simulink library "elementsLibrary"  (R2018a)
settings: Solver=VariableStepAuto  StartTime=0.0  StopTime=10.0  RelTol=1e-3
undefined symbols (not defined in the file): aerodynamics, ascent, avionics, environment, payload, propulsion, pvessel, recovery, rocket, sequencer
libraries: snippetLibrary x43, $bdroot x24, sharedutil x8, theirs_elementsLibrary x3, simulink_extras x1, aerolibutil x1
(part 3 of 4)

== system elementsLibrary/Rocktopus/propulsion ==
  time : Inport
  valveCmd : Inport  Port=2
  temp_atm : Inport  Port=3
  pressure_atm : Inport  Port=4
  "density_atm " : Inport  Port=5
  HREV1 : $bdroot/HREV1  propulsion=rocket.propulsion
  gnd{6..9} (4 alike) : Ground
  thrust_B : Outport
  Ve_gas : Outport  Port=2
  propellantMass : Outport  Port=3
  propellantInertias : Outport  Port=4
  engineProperties : Outport  Port=5
  gasExitSpeed : Outport  Port=6
  motorMass : Outport  Port=7
  motorInertias : Outport  Port=8
  motorGeometry : Outport  Port=9
  wires:
  time/1 -> HREV1/1
  valveCmd/1 -> HREV1/2
  temp_atm/1 -> HREV1/3
  pressure_atm/1 -> HREV1/4
  "density_atm "/1 -> HREV1/5
  HREV1/1 -> thrust_B/1
  HREV1/2 -> Ve_gas/1
  HREV1/3 -> propellantMass/1
  HREV1/4 -> propellantInertias/1
  HREV1/5 -> engineProperties/1
  gnd6/1 -> gasExitSpeed/1
  gnd7/1 -> motorMass/1
  gnd8/1 -> motorInertias/1
  gnd9/1 -> motorGeometry/1

== system elementsLibrary/Rocktopus/recovery ==
  windVelocity : Inport
  density_atm : Inport  Port=2
  envConstants : Inport  Port=3
  inQuaternions : Inport  Port=4
  initVelocity_E : Inport  Port=5
  initPosition_E : Inport  Port=6
  inAngVel : Inport  Port=7
  descentOneDeploy : Inport  Port=8
  descentTwoDeploy : Inport  Port=9
  flightState : Inport  Port=10
  SingleChute : $bdroot/SingleChute  recovery=rocket.recovery
  orientationP : Outport
  angularVelocityP : Outport  Port=2
  angularAccelerationP : Outport  Port=3
  angularAccelerationR : Outport  Port=4
  orientationR : Outport  Port=5
  angularVelocityR : Outport  Port=6
  posP_E : Outport  Port=7
  posR_E : Outport  Port=8
  velocityP_E : Outport  Port=9
  velocityR_E : Outport  Port=10
  accelerationR_E : Outport  Port=11
  accelerationP_E : Outport  Port=12
  wires:
  windVelocity/1 -> SingleChute/1
  density_atm/1 -> SingleChute/2
  envConstants/1 -> SingleChute/3
  inQuaternions/1 -> SingleChute/4
  initVelocity_E/1 -> SingleChute/5
  initPosition_E/1 -> SingleChute/6
  inAngVel/1 -> SingleChute/7
  descentOneDeploy/1 -> SingleChute/8
  descentTwoDeploy/1 -> SingleChute/9
  flightState/1 -> SingleChute/10
  SingleChute/1 -> orientationP/1
  SingleChute/2 -> angularVelocityP/1
  SingleChute/3 -> angularAccelerationP/1
  SingleChute/4 -> angularAccelerationR/1
  SingleChute/5 -> orientationR/1
  SingleChute/6 -> angularVelocityR/1
  SingleChute/7 -> posP_E/1
  SingleChute/8 -> posR_E/1
  SingleChute/9 -> velocityP_E/1
  SingleChute/10 -> velocityR_E/1
  SingleChute/11 -> accelerationR_E/1
  SingleChute/12 -> accelerationP_E/1

== system elementsLibrary/Rocktopus/sequencer ==
  position_E : Inport
  orientation : Inport  Port=2
  velocity_E : Inport  Port=3
  thrust_B : Inport  Port=4
  descentOneDeploy : Inport  Port=5
  descentTwoDeploy : Inport  Port=6
  FSv1 : $bdroot/FSv1  sequencer=rocket.sequencer
  flightState : Outport
  towerVector : Outport  Port=2
  wires:
  position_E/1 -> FSv1/1
  orientation/1 -> FSv1/2
  velocity_E/1 -> FSv1/3
  thrust_B/1 -> FSv1/4
  descentOneDeploy/1 -> FSv1/5
  descentTwoDeploy/1 -> FSv1/6
  FSv1/1 -> flightState/1
  FSv1/2 -> towerVector/1

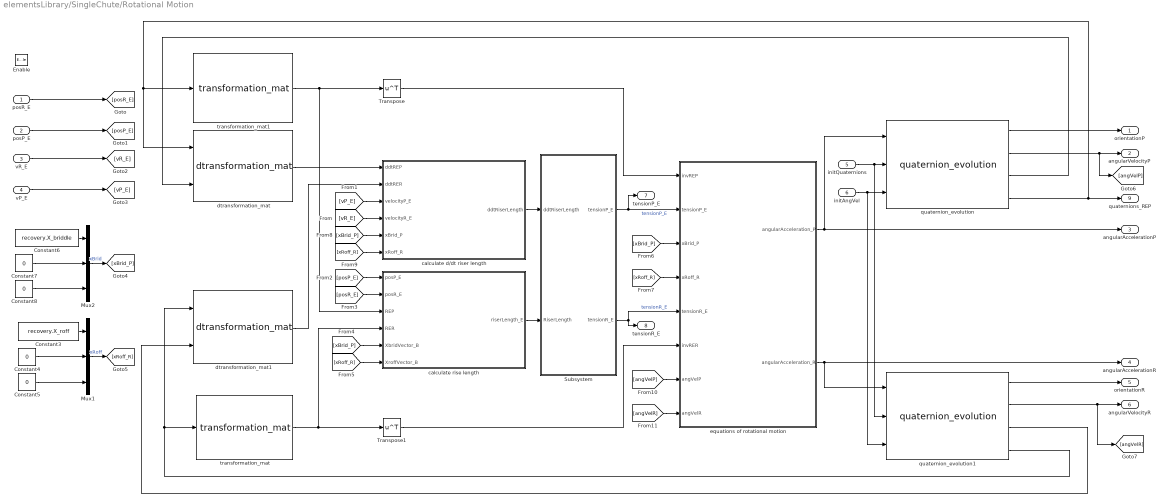
== system elementsLibrary/SingleChute/Rotational Motion ==
  posR_E : Inport
  posP_E : Inport  Port=2
  vR_E : Inport  Port=3
  vP_E : Inport  Port=4
  initQuaternions : Inport  Port=5
  initAngVel : Inport  Port=6
  Enable : EnablePort  StatesWhenEnabling=reset
  Constant3 : Constant  Value=recovery.X_roff
  Constant{4..5,7..8} (4 alike) : Constant  Value=0
  Constant6 : Constant  Value=recovery.X_briddle
  Mux1 : Mux  Inputs=3
  Mux2 : Mux  Inputs=3
  Subsystem : Subsystem
  Transpose : Math  Operator=transpose  SaturateOnIntegerOverflow=on
  Transpose1 : Math  Operator=transpose  SaturateOnIntegerOverflow=on
  calculate d/dt riser length : Subsystem
  calculate rise length : Subsystem
  dtransformation_mat : snippetLibrary/mathSnippets/dtransformation_mat
  dtransformation_mat1 : snippetLibrary/mathSnippets/dtransformation_mat
  equations of rotational motion : Subsystem
  quaternion_evolution : snippetLibrary/mathSnippets/quaternion_evolution
  quaternion_evolution1 : snippetLibrary/mathSnippets/quaternion_evolution
  transformation_mat : snippetLibrary/mathSnippets/transformation_mat
  transformation_mat1 : snippetLibrary/mathSnippets/transformation_mat
  orientationP : Outport
  angularVelocityP : Outport  Port=2
  angularAccelerationP : Outport  Port=3
  angularAccelerationR : Outport  Port=4
  orientationR : Outport  Port=5
  angularVelocityR : Outport  Port=6
  tensionP_E : Outport  Port=7
  tensionR_E : Outport  Port=8
  quaternions_REP : Outport  Port=9
  wires:
  [xRoff_R] -> calculate rise length/6(XroffVector_B)
  equations of rotational motion/2(angularAcceleration_R) -> angularAccelerationR/1, quaternion_evolution1/1
  [posR_E] -> calculate rise length/2(posR_E)
  [posP_E] -> calculate rise length/1(posP_E)
  Constant4/1 -> Mux1/2
  Mux1/1 -> [xRoff_R]  "xRoff"
  posP_E/1 -> [posP_E]
  Subsystem/1(tensionP_E) -> tensionP_E/1, equations of rotational motion/2(tensionP_E)  "tensionP_E"
  calculate d/dt riser length/1(ddtRiserLength) -> Subsystem/1(ddtRiserLength)
  Constant6/1 -> Mux2/1
  calculate rise length/1(riserLength_E) -> Subsystem/2(RiserLength)
  posR_E/1 -> [posR_E]
  [xBrid_P] -> equations of rotational motion/3(xBrid_P)
  [xRoff_R] -> equations of rotational motion/4(xRoff_R)
  [vR_E] -> calculate d/dt riser length/4(velocityR_E)
  Transpose/1 -> equations of rotational motion/1(invREP)
  vP_E/1 -> [vP_E]
  equations of rotational motion/1(angularAcceleration_P) -> angularAccelerationP/1, quaternion_evolution/1
  vR_E/1 -> [vR_E]
  Mux2/1 -> [xBrid_P]  "xBrid"
  Subsystem/2(tensionR_E) -> tensionR_E/1, equations of rotational motion/5(tensionR_E)  "tensionR_E"
  Constant8/1 -> Mux2/3
  Constant3/1 -> Mux1/1
  Constant7/1 -> Mux2/2
  Constant5/1 -> Mux1/3
  [xBrid_P] -> calculate rise length/5(XbridVector_B)
  [vP_E] -> calculate d/dt riser length/3(velocityP_E)
  Transpose1/1 -> equations of rotational motion/6(invRER)
  quaternion_evolution/2 -> angularVelocityP/1, [angVelP]
  quaternion_evolution/1 -> orientationP/1
  quaternion_evolution1/1 -> orientationR/1
  quaternion_evolution1/2 -> [angVelR], angularVelocityR/1
  dtransformation_mat/1 -> calculate d/dt riser length/1(ddtREP)
  transformation_mat1/1 -> Transpose/1, calculate rise length/3(REP)
  transformation_mat/1 -> Transpose1/1, calculate rise length/4(RER)
  quaternion_evolution1/3 -> dtransformation_mat1/2
  quaternion_evolution/3 -> dtransformation_mat/2
  quaternion_evolution1/4 -> transformation_mat/1, dtransformation_mat1/1
  quaternion_evolution/4 -> quaternions_REP/1, transformation_mat1/1, dtransformation_mat/1
  dtransformation_mat1/1 -> calculate d/dt riser length/2(ddtRER)
  [xBrid_P] -> calculate d/dt riser length/5(xBrid_P)
  [xRoff_R] -> calculate d/dt riser length/6(xRoff_R)
  initQuaternions/1 -> quaternion_evolution1/2, quaternion_evolution/2
  [angVelP] -> equations of rotational motion/7(angVelP)
  [angVelR] -> equations of rotational motion/8(angVelR)
  initAngVel/1 -> quaternion_evolution/3, quaternion_evolution1/3

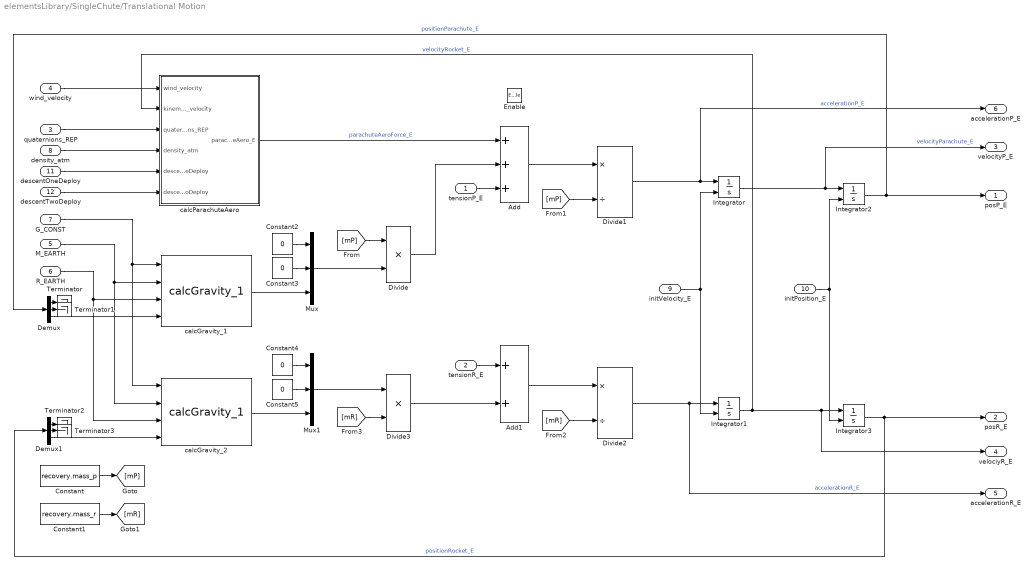
== system elementsLibrary/SingleChute/Translational Motion ==
  tensionP_E : Inport
  tensionR_E : Inport  Port=2
  quaternions_REP : Inport  Port=3
  wind_velocity : Inport  Port=4
  M_EARTH : Inport  Port=5
  R_EARTH : Inport  Port=6
  G_CONST : Inport  Port=7
  density_atm : Inport  Port=8
  initVelocity_E : Inport  Port=9
  initPosition_E : Inport  Port=10
  descentOneDeploy : Inport  Port=11
  descentTwoDeploy : Inport  Port=12
  Enable : EnablePort  StatesWhenEnabling=reset
  Add : Sum  Inputs=+++
  Add1 : Sum
  Constant : Constant  Value=recovery.mass_p
  Constant1 : Constant  Value=recovery.mass_r
  Constant{2..5} (4 alike) : Constant  Value=0
  Demux : Demux  Outputs=3
  Demux1 : Demux  Outputs=3
  Divide : Product  Inputs=**
  Divide1 : Product  Inputs=*/
  Divide2 : Product  Inputs=*/
  Divide3 : Product  Inputs=**
  Integrator{,1..3} (4 alike) : Integrator  InitialConditionSource=external
  Mux : Mux  Inputs=3
  Mux1 : Mux  Inputs=3
  Terminator{,1..3} (4 alike) : Terminator
  calcGravity_1 : snippetLibrary/dynamicsSnippets/calcGravity_1
  calcGravity_2 : snippetLibrary/dynamicsSnippets/calcGravity_1
  "calcParachuteAero " : Subsystem
  posP_E : Outport
  posR_E : Outport  Port=2
  velocityP_E : Outport  Port=3
  velociyR_E : Outport  Port=4
  accelerationR_E : Outport  Port=5
  accelerationP_E : Outport  Port=6
  wires:
  Add1/1 -> Divide2/1
  tensionP_E/1 -> Add/3
  Divide1/1 -> accelerationP_E/1, Integrator/1  "accelerationP_E"
  Integrator/1 -> velocityP_E/1, Integrator2/1  "velocityParachute_E"
  [mP] -> Divide1/2
  Divide2/1 -> accelerationR_E/1, Integrator1/1  "accelerationR_E"
  tensionR_E/1 -> Add1/1
  Add/1 -> Divide1/1
  Constant/1 -> [mP]
  "calcParachuteAero "/1(parachuteAero_E) -> Add/1  "parachuteAeroForce_E"
  [mR] -> Divide2/2
  Divide/1 -> Add/2
  Integrator1/1 -> velociyR_E/1, Integrator3/1, "calcParachuteAero "/2(kinematic_velocity)  "velocityRocket_E"
  Constant1/1 -> [mR]
  Integrator2/1 -> Demux/1, posP_E/1  "positionParachute_E"
  Integrator3/1 -> Demux1/1, posR_E/1  "positionRocket_E"
  quaternions_REP/1 -> "calcParachuteAero "/3(quaternions_REP)
  wind_velocity/1 -> "calcParachuteAero "/1(wind_velocity)
  Divide3/1 -> Add1/2
  [mR] -> Divide3/2
  [mP] -> Divide/1
  Constant2/1 -> Mux/1
  Constant3/1 -> Mux/2
  calcGravity_1/1 -> Mux/3
  Mux/1 -> Divide/2
  calcGravity_2/1 -> Mux1/3
  Mux1/1 -> Divide3/1
  Constant4/1 -> Mux1/1
  Constant5/1 -> Mux1/2
  R_EARTH/1 -> calcGravity_1/3, calcGravity_2/3
  M_EARTH/1 -> calcGravity_1/2, calcGravity_2/2
  G_CONST/1 -> calcGravity_1/1, calcGravity_2/1
  density_atm/1 -> "calcParachuteAero "/4(density_atm)
  Demux/3 -> calcGravity_1/4
  Demux1/3 -> calcGravity_2/4
  initVelocity_E/1 -> Integrator1/2, Integrator/2
  initPosition_E/1 -> Integrator2/2, Integrator3/2
  descentOneDeploy/1 -> "calcParachuteAero "/5(descentOneDeploy)
  descentTwoDeploy/1 -> "calcParachuteAero "/6(descentTwoDeploy)
  Demux1/1 -> Terminator2/1
  Demux1/2 -> Terminator3/1
  Demux/1 -> Terminator/1
  Demux/2 -> Terminator1/1

== system elementsLibrary/SolidMotor/calculate motor inertia ==
  motorMass : Inport
  grainInnerDia : Inport  Port=2
  grainOuterDia : Inport  Port=3
  grainLength : Inport  Port=4
  Add : Sum
  Add1 : Sum
  Constant{,1..5} (6 alike) : Constant  Value=0
  Create 3x3 Matrix : sharedutil/Create 3x3 Matrix  aMode=aMode
  Gain : Gain  Gain=0.5
  Gain1 : Gain  Gain=0.5
  Gain2 : Gain  Gain=3
  Gain3 : Gain  Gain=1/12
  Gain4 : Gain  Gain=0.5
  Gain5 : Gain
  Multiply : Product
  Multiply1 : Product
  Square : Math  Operator=square  SaturateOnIntegerOverflow=on
  Square1 : Math  Operator=square  SaturateOnIntegerOverflow=on
  Square2 : Math  Operator=square  SaturateOnIntegerOverflow=on
  J_motor : Outport
  wires:
  Create 3x3 Matrix/1 -> J_motor/1  "inertias"
  grainLength/1 -> Square2/1
  grainInnerDia/1 -> Gain/1
  Gain/1 -> Square/1
  grainOuterDia/1 -> Gain1/1
  Gain1/1 -> Square1/1
  Square/1 -> Add/1
  Square1/1 -> Add/2
  Add/1 -> Multiply1/1, Gain2/1
  Gain2/1 -> Add1/1
  Square2/1 -> Add1/2
  motorMass/1 -> Gain3/1
  Add1/1 -> Multiply/1
  Gain3/1 -> Multiply1/2, Multiply/2
  Multiply/1 -> Create 3x3 Matrix/9, Gain5/1  "Izz"
  Multiply1/1 -> Gain4/1
  Gain4/1 -> Create 3x3 Matrix/1  "Ixx"
  Gain5/1 -> Create 3x3 Matrix/5  "Iyy"
  Constant/1 -> Create 3x3 Matrix/2
  Constant1/1 -> Create 3x3 Matrix/3
  Constant2/1 -> Create 3x3 Matrix/4
  Constant3/1 -> Create 3x3 Matrix/6
  Constant4/1 -> Create 3x3 Matrix/7
  Constant5/1 -> Create 3x3 Matrix/8

== system elementsLibrary/barrowmanExt/CalcMach ==
  Temperatue_atm : Inport
  kinematicVelocity : Inport  Port=2
  Add : Sum
  Constant : Constant  Value=20.05
  Constant1 : Constant  Value=273.1
  Divide : Product  Inputs=*/
  Multiply : Product
  Sqrt : Sqrt  SaturateOnIntegerOverflow=on
  magnitude_3 : snippetLibrary/mathSnippets/magnitude_3
  Mach : Outport
  wires:
  Temperatue_atm/1 -> Add/2
  Constant1/1 -> Add/1
  Add/1 -> Sqrt/1
  Constant/1 -> Multiply/2
  Sqrt/1 -> Multiply/1
  Multiply/1 -> Divide/2
  Divide/1 -> Mach/1
  kinematicVelocity/1 -> magnitude_3/1
  magnitude_3/1 -> Divide/1

== system elementsLibrary/barrowmanExt/Center of Pressure ==
  Cna_body : Inport
  Cna_fins : Inport  Port=2
  Cna_nosecone : Inport  Port=3
  Mach : Inport  Port=4
  Add : Sum  Inputs=+++
  Add1 : Sum  Inputs=+++
  Calc Xcp fins : Subsystem
  Constant : Constant  Value=aerodynamics.Xcp_nose
  Constant2 : Constant  Value=aerodynamics.Xcp_body
  Divide : Product  Inputs=*/
  Multiply : Product
  Multiply1 : Product
  Multiply2 : Product
  Xcp : Outport
  wires:
  Constant/1 -> Multiply/2
  Cna_nosecone/1 -> Add1/3, Multiply/1
  Cna_fins/1 -> Add1/2, Multiply2/1
  Constant2/1 -> Multiply1/1
  Cna_body/1 -> Add1/1, Multiply1/2
  Multiply/1 -> Add/3
  Multiply2/1 -> Add/2
  Multiply1/1 -> Add/1
  Add/1 -> Divide/1
  Add1/1 -> Divide/2
  Divide/1 -> Xcp/1
  Calc Xcp fins/1(Xcp_fins) -> Multiply2/2
  Mach/1 -> Calc Xcp fins/1(Mach)

== system elementsLibrary/barrowmanExt/Coeff multiplier ==
  Velocity_B : Inport
  Density_air : Inport  Port=2
  Constant : Constant  Value=0.5
  Constant1 : Constant  Value=aerodynamics.Ar
  Multiply : Product  Inputs=4
  Square : Math  Operator=square  SaturateOnIntegerOverflow=on
  magnitude_3 : Subsystem
  Coeff_mul : Outport
  wires:
  Velocity_B/1 -> magnitude_3/1(vector)
  magnitude_3/1(magnitude) -> Square/1
  Square/1 -> Multiply/1
  Density_air/1 -> Multiply/2
  Constant/1 -> Multiply/3
  Constant1/1 -> Multiply/4
  Multiply/1 -> Coeff_mul/1

== system elementsLibrary/barrowmanExt/Coeff multiplier1 ==
  Velocity_B : Inport
  Density_air : Inport  Port=2
  Constant : Constant  Value=0.5
  Constant1 : Constant  Value=aerodynamics.Ar
  Constant2 : Constant  Value=aerodynamics.dn
  Multiply : Product  Inputs=5
  Square : Math  Operator=square  SaturateOnIntegerOverflow=on
  magnitude_3 : Subsystem
  Coeff_mul : Outport
  wires:
  Velocity_B/1 -> magnitude_3/1(vector)
  magnitude_3/1(magnitude) -> Square/1
  Square/1 -> Multiply/1
  Density_air/1 -> Multiply/2
  Constant/1 -> Multiply/3
  Constant1/1 -> Multiply/4
  Multiply/1 -> Coeff_mul/1
  Constant2/1 -> Multiply/5

== system elementsLibrary/barrowmanExt/Coefficent of drag 0 AOA ==
  Mach : Inport
  RE_Body : Inport  Port=2
  RE_Fins : Inport  Port=3
  Add : Sum  Inputs=+++
  Base Drag Coefficient : Subsystem
  Friction Drag Coefficient : Subsystem
  Pressure Drag Coefficient : Subsystem
  Cd_0 : Outport
  wires:
  RE_Body/1 -> Friction Drag Coefficient/2(RE_Body)
  RE_Fins/1 -> Friction Drag Coefficient/3(RE_Fins)
  Mach/1 -> Pressure Drag Coefficient/2(mach), Friction Drag Coefficient/1(mach), Base Drag Coefficient/1(Mach)
  Base Drag Coefficient/1(Cd_Base) -> Add/1, Pressure Drag Coefficient/1(Cd_Base)
  Pressure Drag Coefficient/1(Cd_Pressure) -> Add/2
  Friction Drag Coefficient/1(CD_Friction) -> Add/3
  Add/1 -> Cd_0/1

== system elementsLibrary/barrowmanExt/Coefficient of Axial Force ==
  AOA : Inport
  Cd_0 : Inport  Port=2
  If : If  IfExpression=u1 <=0.2967
  If Action Subsystem : Subsystem  TreatAsAtomicUnit=on
  If Action Subsystem1 : Subsystem  TreatAsAtomicUnit=on
  If Action Subsystem2 : Subsystem  TreatAsAtomicUnit=on
  If Action Subsystem3 : Subsystem  TreatAsAtomicUnit=on
  If Action Subsystem4 : Subsystem  TreatAsAtomicUnit=on
  If Action Subsystem5 : Subsystem  TreatAsAtomicUnit=on
  If1 : If  IfExpression=u1 > 1.5708
  If2 : If  IfExpression=u1 > 1.5708
  Merge : Merge
  Merge1 : Merge
  Merge2 : Merge
  Multiply : Product
  Cax : Outport
  wires:
  If/1 -> If Action Subsystem/Action
  AOA/1 -> If2/1, If Action Subsystem2/1(AOA_init), If Action Subsystem1/1(AOA_init), If1/1
  If1/1 -> If Action Subsystem1/Action
  If1/2 -> If Action Subsystem2/Action
  If Action Subsystem2/1(AOA) -> Merge/2
  If Action Subsystem1/1(AOA) -> Merge/1
  Merge/1 -> If Action Subsystem3/1(AOA), If/1, If Action Subsystem/1(AOA)
  If/2 -> If Action Subsystem3/Action
  If Action Subsystem/1(Ax_multi) -> Merge1/1
  If Action Subsystem3/1(Ax_multi) -> Merge1/2
  If2/1 -> If Action Subsystem4/Action
  If2/2 -> If Action Subsystem5/Action
  Merge1/1 -> If Action Subsystem4/1(Ax_multi_init), If Action Subsystem5/1(Ax_multi_init)
  If Action Subsystem4/1(Ax_multi) -> Merge2/1
  If Action Subsystem5/1(Ax_multi) -> Merge2/2
  Merge2/1 -> Multiply/2
  Cd_0/1 -> Multiply/1
  Multiply/1 -> Cax/1

== system elementsLibrary/barrowmanExt/Coefficient of normal force ==
  k1 : Inport
  k2 : Inport  Port=2
  k3 : Inport  Port=3
  Mach : Inport  Port=4
  AOA : Inport  Port=5
  Add : Sum
  Add1 : Sum
  Body tube correction : Subsystem
  Cna Body Tube : Subsystem
  Cna Fins : Subsystem
  Divide : Product  Inputs=*/
  Multiply : Product
  Cn : Outport
  Cna_body : Outport  Port=2
  Cna_fins : Outport  Port=3
  Cna_nosecone : Outport  Port=4
  wires:
  AOA/1 -> Cna Fins/1(AOA), Body tube correction/1(AOA), Divide/2, Multiply/1, Cna Body Tube/1(AOA)
  Mach/1 -> Cna Fins/2(Mach)
  k1/1 -> Cna Fins/3(k1)
  k2/1 -> Cna Fins/4(k2)
  k3/1 -> Cna Fins/5(k3)
  Cna Body Tube/1(Cna_nosecone) -> Cna_nosecone/1, Add/1
  Cna Fins/1(Cna_fins_w_FB_inter) -> Cna_fins/1, Add/2
  Add/1 -> Multiply/2
  Body tube correction/1(Cn_BodyCorrection) -> Divide/1, Add1/1
  Multiply/1 -> Add1/2
  Add1/1 -> Cn/1
  Divide/1 -> Cna_body/1

== system elementsLibrary/barrowmanExt/Moment Coefficients from nosetip ==
  Xcp : Inport
  Cn : Inport  Port=2
  rollAngle : Inport  Port=3
  Xcg : Inport  Port=4
  Constant1 : Constant  Value=0
  Cos : Trigonometry  Operator=cos
  Multiply : Product
  Multiply1 : Product
  Pitch Moment Coeff : Subsystem
  Sin : Trigonometry
  Subsystem : Subsystem
  Cm_roll : Outport
  Cm_pitch : Outport  Port=2
  Cm_yaw : Outport  Port=3
  wires:
  Xcp/1 -> Pitch Moment Coeff/1(Xcp)
  Cn/1 -> Subsystem/2(Cn), Pitch Moment Coeff/2(Cn)
  Pitch Moment Coeff/1(Cm_pitch_cp) -> Subsystem/1(Cm_pitch_cp)
  Xcg/1 -> Subsystem/3(Xcg)
  Cos/1 -> Multiply/1
  Multiply1/1 -> Cm_yaw/1
  Multiply/1 -> Cm_pitch/1
  rollAngle/1 -> Cos/1, Sin/1
  Subsystem/1(Cm_pitch_cg) -> Multiply1/1, Multiply/2
  Sin/1 -> Multiply1/2
  Constant1/1 -> Cm_roll/1

== system elementsLibrary/barrowmanExt/Reynolds num ==
  Velocity : Inport
  Kinematic Viscosity : Inport  Port=2
  Constant : Constant  Value=aerodynamics.l_TR
  Constant1 : Constant  Value=aerodynamics.lm
  Divide : Product  Inputs=*/
  Multiply : Product
  Multiply1 : Product
  magnitude_3 : snippetLibrary/mathSnippets/magnitude_3
  Reynolds_Body : Outport
  Reynolds_Fins : Outport  Port=2
  wires:
  Kinematic Viscosity/1 -> Divide/2
  Multiply/1 -> Reynolds_Body/1
  Constant/1 -> Multiply/1
  Divide/1 -> Multiply1/1, Multiply/2
  Multiply1/1 -> Reynolds_Fins/1
  Constant1/1 -> Multiply1/2
  Velocity/1 -> magnitude_3/1
  magnitude_3/1 -> Divide/1

== system elementsLibrary/nitrousTank1/Nitrous_Inertia_and_cg ==
  mass : Inport
  density : Inport  Port=2
  Add : Sum
  Constant{,1..6} (7 alike) : Constant  Value=0
  Constant10 : Constant  Value=pvessel.L_OxiTank
  Constant7 : Constant  Value=pi
  Constant8 : Constant  Value=2
  Constant9 : Constant  Value=pvessel.D_OxiTank
  Create 3x3 Matrix : sharedutil/Create 3x3 Matrix  aMode=aMode
  Divide : Product  Inputs=*/
  Divide1 : Product  Inputs=*/
  Divide2 : Product  Inputs=*/
  Gain : Gain  Gain=1/12
  Gain1 : Gain  Gain=1/2
  Gain2 : Gain  Gain=3
  Gain3 : Gain  Gain=1/2
  Multiply : Product
  Multiply1 : Product
  Square : Math  Operator=square  SaturateOnIntegerOverflow=on
  Square1 : Math  Operator=square  SaturateOnIntegerOverflow=on
  Square2 : Math  Operator=square  SaturateOnIntegerOverflow=on
  Terminator : Terminator
  Inertia_oxi : Outport
  X_cg : Outport  Port=2
  wires:
  Constant9/1 -> Gain3/1, Gain1/1
  Gain1/1 -> Square1/1
  Square1/1 -> Gain2/1
  Square/1 -> Add/1
  Gain2/1 -> Add/2
  Gain/1 -> Multiply/1
  Add/1 -> Multiply/2
  Multiply/1 -> Create 3x3 Matrix/4, Create 3x3 Matrix/9
  Constant/1 -> Create 3x3 Matrix/2
  Constant1/1 -> Create 3x3 Matrix/1
  Constant2/1 -> Create 3x3 Matrix/3
  Constant3/1 -> Create 3x3 Matrix/5
  Constant4/1 -> Create 3x3 Matrix/6
  Constant5/1 -> Create 3x3 Matrix/7
  Constant6/1 -> Create 3x3 Matrix/8
  Create 3x3 Matrix/1 -> Inertia_oxi/1
  Gain3/1 -> Square2/1  "r_oxi"
  Square2/1 -> Multiply1/2
  Divide2/1 -> Divide/1, Square/1  "h_oxi"
  Constant8/1 -> Divide/2
  Divide1/1 -> Divide2/1  "Volume_oxi"
  density/1 -> Divide1/2
  mass/1 -> Divide1/1, Gain/1  "mass_oxi"
  Multiply1/1 -> Divide2/2  "Pi*(r2)"
  Constant7/1 -> Multiply1/1
  Divide/1 -> X_cg/1
  Constant10/1 -> Terminator/1

== system elementsLibrary/Ascentv1/Calculate Aero Coeffs & Center of Pressure/calculate AOA & Side Slip ==
  apparentVelocity_B : Inport
  calcAoA : MATLAB Function  TreatAsAtomicUnit=on
  AOA : Outport
  aeroRollAngle : Outport  Port=2
  wires:
  calcAoA/1(alpha) -> AOA/1
  apparentVelocity_B/1 -> calcAoA/1(Va)
  calcAoA/2(phiA) -> aeroRollAngle/1

== system elementsLibrary/Ascentv1/Calculate Aero Coeffs & Center of Pressure/calculate Mach ==
  temperature_atm : Inport
  apparentVelocity_E : Inport  Port=2
  Add : Sum
  Constant : Constant  Value=331.3
  Constant1 : Constant  Value=0.606
  Divide : Product  Inputs=*/
  Multiply : Product
  magnitude_3 : snippetLibrary/mathSnippets/magnitude_3
  mach : Outport
  speed of sound : Outport  Port=2
  wires:
  Constant1/1 -> Multiply/2
  Multiply/1 -> Add/1
  Constant/1 -> Add/2
  Add/1 -> Divide/2, speed of sound/1  "speedOfSound"
  Divide/1 -> mach/1  "mach"
  apparentVelocity_E/1 -> magnitude_3/1
  magnitude_3/1 -> Divide/1  "VaMag_B"
  temperature_atm/1 -> Multiply/1

== system elementsLibrary/Ascentv1/Calculate Aero Coeffs & Center of Pressure/calculate ZAOA_cd ==
  note: Calculating Relavent Reynolds Number
  apparentVelocity_B : Inport
  density_atm : Inport  Port=2
  kinViscosity_atm : Inport  Port=3
  Add : Sum  Inputs=++++
  BaseCd : Subsystem
  Constant : Constant  Value=ascent.aerodynamics.l_TR
  Constant1 : Constant  Value=ascent.aerodynamics.lm
  Constant2 : Constant  Value=ascent.aerodynamics.REC
  Divide : Product  Inputs=*/
  FinsetCd : Subsystem
  ForebodyCd : Subsystem
  InterferenceCd : Subsystem
  MATLAB Function : snippetLibrary/aeroSnippets/MATLAB Function
  MATLAB Function1 : snippetLibrary/aeroSnippets/MATLAB Function
  Multiply1 : Product
  Multiply2 : Product
  Terminator : Terminator
  magnitude_3 : snippetLibrary/mathSnippets/magnitude_3
  ZAOA_cd : Outport
  wires:
  magnitude_3/1 -> Divide/1
  Divide/1 -> Multiply1/2, Multiply2/1
  Constant/1 -> Multiply1/1
  Constant1/1 -> Multiply2/2
  Multiply1/1 -> MATLAB Function/1  "reynoldBody"
  Multiply2/1 -> MATLAB Function1/1  "reynoldFinSet"
  Constant2/1 -> MATLAB Function1/2, MATLAB Function/2
  MATLAB Function/1 -> ForebodyCd/1(Cf_fb)  "cf_fb"
  MATLAB Function1/1 -> InterferenceCd/1(Cf_f), FinsetCd/1(Cf_f)  "cf_f"
  FinsetCd/1(Cdf) -> Add/4  "Cdf"
  Add/1 -> ZAOA_cd/1  "ZAOA_cd"
  ForebodyCd/1(Cd_fb) -> Add/1, BaseCd/1(Cd_fb)  "Cd_fb"
  BaseCd/1(Cdb) -> Add/2
  InterferenceCd/1(Cdi) -> Add/3  "Cdi"
  kinViscosity_atm/1 -> Divide/2
  apparentVelocity_B/1 -> magnitude_3/1
  density_atm/1 -> Terminator/1

== system elementsLibrary/Ascentv1/Rotation/Subsystem ==
  angVel : Inport
  sumOfMoments : Inport  Port=2
  J_rocket : Inport  Port=3
  Add : Sum  Inputs=-+
  Matrix Multiply : Product  Inputs=/*  Multiplication=Matrix(*)
  Matrix Multiply2 : Product  Multiplication=Matrix(*)
  crossProduct : snippetLibrary/mathSnippets/crossProduct
  angularAcceleration : Outport
  wires:
  crossProduct/1 -> Add/1
  Matrix Multiply2/1 -> crossProduct/2
  Add/1 -> Matrix Multiply/2
  Matrix Multiply/1 -> angularAcceleration/1  "angularAcceleration"
  angVel/1 -> crossProduct/1, Matrix Multiply2/2
  J_rocket/1 -> Matrix Multiply/1, Matrix Multiply2/1
  sumOfMoments/1 -> Add/2

== system elementsLibrary/Ascentv1/Rotation/momentCalculation ==
  Fthrust_B : Inport
  Faero_B : Inport  Port=2
  Xcg : Inport  Port=3
  Xcp : Inport  Port=4
  Constant : Constant  Value=ascent.aerodynamics.l_TR
  Constant{1..5} (5 alike) : Constant  Value=0
  Mux : Mux  Inputs=3
  Mux1 : Mux  Inputs=3
  Mux2 : Mux  Inputs=3
  Subtract : Sum  Inputs=-+
  Subtract1 : Sum  Inputs=-+
  Terminator : Terminator
  Terminator1 : Terminator
  crossProduct : snippetLibrary/mathSnippets/crossProduct
  crossProduct1 : snippetLibrary/mathSnippets/crossProduct
  momentsAero : Outport
  momentsThrust : Outport  Port=2
  wires:
  Xcp/1 -> Subtract/1
  Xcg/1 -> Subtract1/2, Subtract/2
  Constant/1 -> Subtract1/1
  Subtract/1 -> Mux/1  "rsm"
  Constant1/1 -> Mux/2
  Constant2/1 -> Mux/3
  Constant3/1 -> Mux1/2
  Constant4/1 -> Mux1/3
  Mux/1 -> crossProduct/1
  Mux1/1 -> crossProduct1/1
  Faero_B/1 -> crossProduct/2
  Fthrust_B/1 -> crossProduct1/2
  Subtract1/1 -> Mux1/1  "rcgm"
  Constant5/1 -> Mux2/3, Mux2/2, Mux2/1
  Mux2/1 -> Terminator1/1
  crossProduct1/1 -> momentsThrust/1
  crossProduct/1 -> momentsAero/1

== system elementsLibrary/Ascentv1/Rotation/momentDamping ==
  angularVel_B : Inport
  apparentVelocity : Inport  Port=2
  mach : Inport  Port=3
  density_atm : Inport  Port=4
  xcg : Inport  Port=5
  Constant : Constant  Value=ascent.aerodynamics.Xf
  Constant1 : Constant  Value=ascent.aerodynamics.lt
  Constant10 : Constant  Value=ascent.aerodynamics.nf
  Constant2 : Constant  Value=ascent.aerodynamics.lr
  Constant3 : Constant  Value=ascent.aerodynamics.df/2
  Constant4 : Constant  Value=ascent.aerodynamics.ls
  Constant5 : Constant  Value=ascent.aerodynamics.lw
  Constant6 : Constant  Value=ascent.aerodynamics.l_TR
  Constant7 : Constant  Value=ascent.aerodynamics.dn
  Constant8 : Constant  Value=ascent.aerodynamics.Ar
  Constant9 : Constant  Value=ascent.aerodynamics.deq
  calcMomentDamping : MATLAB Function  TreatAsAtomicUnit=on
  rollDampingMoment : Outport
  pitchDampingMoment : Outport  Port=2
  yawDampingMoment : Outport  Port=3
  wires:
  apparentVelocity/1 -> calcMomentDamping/1(Va)
  angularVel_B/1 -> calcMomentDamping/2(angVel)
  mach/1 -> calcMomentDamping/3(mach)
  density_atm/1 -> calcMomentDamping/4(density_atm)
  Constant1/1 -> calcMomentDamping/7(ct)
  Constant6/1 -> calcMomentDamping/12(l_TR)
  Constant7/1 -> calcMomentDamping/13(l_ref)
  Constant8/1 -> calcMomentDamping/14(A_ref)
  Constant9/1 -> calcMomentDamping/15(Deq)
  Constant10/1 -> calcMomentDamping/16(numFins)
  calcMomentDamping/1(Mx_damp) -> rollDampingMoment/1
  calcMomentDamping/2(My_damp) -> pitchDampingMoment/1
  calcMomentDamping/3(Mz_damp) -> yawDampingMoment/1
  xcg/1 -> calcMomentDamping/5(xcg)
  Constant/1 -> calcMomentDamping/6(X_finset)
  Constant5/1 -> calcMomentDamping/11(w)
  Constant4/1 -> calcMomentDamping/10(s)
  Constant3/1 -> calcMomentDamping/9(rt)
  Constant2/1 -> calcMomentDamping/8(cr)

== system elementsLibrary/Ascentv2/Rotational/Inertia_Matrix  ==
  motorInertias : Inport
  propellantMass : Inport  Port=2
  motorProperties : Inport  Port=3
  rocketEmptyXcg : Inport  Port=4
  Constant : Constant  Value=ascent.InertiaMatNoEngine
  parallelAxisTheo_restricted : Subsystem
  J_rocket : Outport
  wires:
  parallelAxisTheo_restricted/1(J_rocket) -> J_rocket/1
  Constant/1 -> parallelAxisTheo_restricted/1(emptyInertia)
  motorInertias/1 -> parallelAxisTheo_restricted/2(motorInertias)
  propellantMass/1 -> parallelAxisTheo_restricted/3(propellantMass)
  rocketEmptyXcg/1 -> parallelAxisTheo_restricted/4(rocketEmptyXcg)
  motorProperties/1 -> parallelAxisTheo_restricted/5(motorProperties)

== system elementsLibrary/Ascentv2/Rotational/Subsystem ==
  angVel : Inport
  J_rocket : Inport  Port=2
  sumOfMoments : Inport  Port=3
  Add : Sum  Inputs=-+
  Matrix Multiply : Product  Inputs=/*  Multiplication=Matrix(*)
  Matrix Multiply2 : Product  Multiplication=Matrix(*)
  crossProduct : snippetLibrary/mathSnippets/crossProduct
  angularAcceleration : Outport
  wires:
  Matrix Multiply2/1 -> crossProduct/2
  crossProduct/1 -> Add/1
  Add/1 -> Matrix Multiply/2
  Matrix Multiply/1 -> angularAcceleration/1  "angularAcceleration"
  J_rocket/1 -> Matrix Multiply/1, Matrix Multiply2/1
  sumOfMoments/1 -> Add/2
  angVel/1 -> crossProduct/1, Matrix Multiply2/2

== system elementsLibrary/Ascentv2/Rotational/quaternion_evolution ==
  angularAccelerations_B : Inport
  initialQuaternions : Inport  Port=2
  initialAngVel : Inport  Port=3
  Calculate Euler Triplet from Quaternion : MATLAB Function  TreatAsAtomicUnit=on
  Calculate Rate of Change of Quaternions : MATLAB Function  TreatAsAtomicUnit=on
  Constant : Constant  Value=0
  Integrator : Integrator  InitialConditionSource=external
  Integrator1 : Integrator  InitialConditionSource=external  InitialCondition=[1;1;1;1]
  Terminator : Terminator
  euler_angles : Outport
  anguarVelocity : Outport  Port=2
  ddtQuaternions : Outport  Port=3
  quaternions : Outport  Port=4
  wires:
  Integrator1/1 -> Calculate Euler Triplet from Quaternion/1(Quaternions), Calculate Rate of Change of Quaternions/2(Quaternions), quaternions/1
  Calculate Euler Triplet from Quaternion/1(euler_angles) -> euler_angles/1
  Calculate Rate of Change of Quaternions/1(ddt_Quaternions) -> ddtQuaternions/1, Integrator1/1
  initialQuaternions/1 -> Integrator1/2  "initial quaternions"
  Integrator/1 -> Calculate Rate of Change of Quaternions/1(angularVelocities_B), anguarVelocity/1
  initialAngVel/1 -> Integrator/2
  angularAccelerations_B/1 -> Terminator/1
  Constant/1 -> Integrator/1

== system elementsLibrary/HREV1/Chamber_Ballistics/Inertia ==
  massFuel : Inport
  Grain_inner_dia : Inport  Port=2
  Grain_outer_dia : Inport  Port=3
  X_fuel_length : Inport  Port=4
  Add : Sum
  Add1 : Sum
  Constant{,1..6} (7 alike) : Constant  Value=0
  Create 3x3 Matrix : sharedutil/Create 3x3 Matrix  aMode=aMode
  Gain : Gain  Gain=1/12
  Gain1 : Gain  Gain=1/2
  Gain2 : Gain  Gain=1/2
  Gain3 : Gain  Gain=3
  Multiply : Product
  Square : Math  Operator=square  SaturateOnIntegerOverflow=on
  Square1 : Math  Operator=square  SaturateOnIntegerOverflow=on
  Square2 : Math  Operator=square  SaturateOnIntegerOverflow=on
  Fuel_inertia : Outport
  wires:
  massFuel/1 -> Gain/1
  Gain/1 -> Multiply/1
  Add/1 -> Gain3/1
  Gain3/1 -> Add1/1
  Gain1/1 -> Square1/1
  Square1/1 -> Add/1
  Gain2/1 -> Square2/1
  Square2/1 -> Add/2
  X_fuel_length/1 -> Square/1
  Square/1 -> Add1/2
  Add1/1 -> Multiply/2
  Constant5/1 -> Create 3x3 Matrix/5
  Multiply/1 -> Create 3x3 Matrix/4, Create 3x3 Matrix/9
  Create 3x3 Matrix/1 -> Fuel_inertia/1
  Constant/1 -> Create 3x3 Matrix/1
  Constant1/1 -> Create 3x3 Matrix/2
  Constant2/1 -> Create 3x3 Matrix/3
  Constant6/1 -> Create 3x3 Matrix/6
  Constant3/1 -> Create 3x3 Matrix/7
  Constant4/1 -> Create 3x3 Matrix/8
  Grain_inner_dia/1 -> Gain2/1
  Grain_outer_dia/1 -> Gain1/1

== system elementsLibrary/HREV1/Chamber_Ballistics/calc_chamber_params ==
  OF_ratio : Inport
  mdot_prop : Inport  Port=2
  cStar : Inport  Port=3
  A_throat : Constant  Value=propulsion.At
  Constant : Constant  Value=101.325
  Divide : Product  Inputs=*/
  If : If  IfExpression=u1 >= 101.325
  If Action Subsystem : Subsystem  TreatAsAtomicUnit=on
  If Action Subsystem1 : Subsystem  TreatAsAtomicUnit=on
  Merge : Merge
  Multiply : Product
  Pa_to_kPa : Gain  Gain=0.001
  calc_Tc : Subsystem
  Pc : Outport
  Tc : Outport  Port=2
  wires:
  OF_ratio/1 -> calc_Tc/1(OF_ratio)
  calc_Tc/1(Tc) -> Tc/1
  Divide/1 -> Pa_to_kPa/1
  Multiply/1 -> Divide/1
  A_throat/1 -> Divide/2
  mdot_prop/1 -> Multiply/1
  cStar/1 -> Multiply/2
  If Action Subsystem/1(Out1) -> Merge/1
  Constant/1 -> If Action Subsystem1/1(In1)
  If/2 -> If Action Subsystem1/Action
  Merge/1 -> Pc/1
  If/1 -> If Action Subsystem/Action
  If Action Subsystem1/1(Out1) -> Merge/2
  Pa_to_kPa/1 -> If/1, If Action Subsystem/1(In1)

== system elementsLibrary/HREV1/Chamber_Ballistics/calc_mdot_fuel ==
  mdot_oxi : Inport
  Dp : Inport  Port=2
  Constant : Constant  Value=propulsion.rho_fuel
  calc_OF : Subsystem
  calc_massFlux_oxi : Subsystem
  calc_mdot_fuel : Subsystem
  calc_rdot_fuel : Subsystem
  Gox : Outport
  rdot_f : Outport  Port=2
  mdot_f : Outport  Port=3
  OF_ratio : Outport  Port=4
  massFuel : Outport  Port=5
  wires:
  Dp/1 -> calc_mdot_fuel/2(Dp), calc_massFlux_oxi/1(Dp)
  mdot_oxi/1 -> calc_OF/2(mdot_oxi), calc_massFlux_oxi/2(mdot_oxi)
  calc_massFlux_oxi/1(Gox) -> Gox/1, calc_rdot_fuel/1(Gox)
  calc_rdot_fuel/1(rdot_fuel) -> calc_mdot_fuel/1(rdot_fuel), rdot_f/1
  calc_mdot_fuel/1(mdot_fuel) -> calc_OF/1(mdot_fuel), mdot_f/1
  calc_OF/1(OF_ratio) -> OF_ratio/1
  Constant/1 -> calc_mdot_fuel/3(rho_oxi)
  calc_mdot_fuel/2(massFuel) -> massFuel/1

== system elementsLibrary/HREV1/Chamber_Ballistics/calc_port_diameter ==
  note: another way to compute dDp_dt?
  mdot_oxi : Inport
  Dp_prev : Inport  Port=2
  rdot_f : Inport  Port=3
  Add : Sum  Commented=on
  Constant : Constant  Commented=on  Value=2
  Constant1 : Constant  Commented=on
  Divide : Product  Commented=on  Inputs=*/
  Divide1 : Product  Commented=on  Inputs=*/
  Gain : Gain  Commented=on  Gain=2
  Gain1 : Gain  Gain=2
  Less Than : RelationalOperator  Operator=<  OutDataTypeStr=boolean  RndMeth=Simplest
  Multiply : Product  Commented=on
  Multiply1 : Product  Commented=on
  Multiply2 : Product
  Pi : Constant  Commented=on  Value=pi
  Power{,1..3} (4 alike) : Math  Commented=on  Operator=pow  SaturateOnIntegerOverflow=on
  Terminator : Terminator  Commented=on
  a : Constant  Commented=on  Value=propulsion.a
  n : Constant  Commented=on  Value=propulsion.n
  outer_grain_diameter : Constant  Value=propulsion.Dfg_outer
  dDp_dt : Outport
  wires:
  Multiply/1 -> Terminator/1
  Divide/1 -> Multiply/1
  Divide1/1 -> Multiply/2
  Power1/1 -> Divide/2
  Pi/1 -> Power1/1
  Multiply1/1 -> Divide/1
  Power/1 -> Multiply1/1
  a/1 -> Multiply1/2
  Add/1 -> Power/2
  n/1 -> Power2/2, Power1/2, Gain/1
  Constant/1 -> Power/1
  Gain/1 -> Power3/2, Add/1
  Constant1/1 -> Add/2
  Power2/1 -> Divide1/1
  mdot_oxi/1 -> Power2/1
  Power3/1 -> Divide1/2
  outer_grain_diameter/1 -> Less Than/2
  Less Than/1 -> Multiply2/2
  Multiply2/1 -> dDp_dt/1
  Dp_prev/1 -> Power3/1, Less Than/1
  rdot_f/1 -> Gain1/1
  Gain1/1 -> Multiply2/1

== system elementsLibrary/HREV1/Nozzle/calc_Vexit ==
  Tc : Inport
  Pc : Inport  Port=2
  Pe : Inport  Port=3
  Constant : Constant  Value=propulsion.gasConst
  Constant1 : Constant
  Constant2 : Constant  Value=propulsion.k - 1
  Constant3 : Constant  Value=propulsion.k
  Divide : Product  Inputs=*/
  Divide1 : Product  Inputs=*/
  Divide2 : Product  Inputs=*/
  Gain : Gain  Gain=2
  Multiply : Product
  Multiply1 : Product  Inputs=3
  Power : Math  Operator=pow  SaturateOnIntegerOverflow=on
  Sqrt : Sqrt  SaturateOnIntegerOverflow=on
  Subtract : Sum  Inputs=+-
  Ve_gas : Outport
  wires:
  Sqrt/1 -> Ve_gas/1
  Multiply/1 -> Sqrt/1
  Subtract/1 -> Multiply/2
  Constant1/1 -> Subtract/1
  Power/1 -> Subtract/2
  Divide/1 -> Power/1
  Pe/1 -> Divide/1
  Pc/1 -> Divide/2
  Divide1/1 -> Power/2
  Constant2/1 -> Divide2/2, Divide1/1
  Constant3/1 -> Multiply1/3, Divide1/2
  Divide2/1 -> Multiply/1
  Gain/1 -> Divide2/1
  Multiply1/1 -> Gain/1
  Constant/1 -> Multiply1/2
  Tc/1 -> Multiply1/1

== system elementsLibrary/HREV1/Nozzle/calc_charVel ==
  speedOfSound : Inport
  Combustion Efficiency : Constant  Value=propulsion.etaCombustion
  Combustion Efficiency1 : Constant  Value=propulsion.k + 1
  Combustion Efficiency2 : Constant  Value=2*propulsion.k - 2
  Constant : Constant  Value=2
  Divide : Product  Inputs=*/
  Divide1 : Product  Inputs=*/
  Divide2 : Product  Inputs=*/
  Gain : Gain  Gain=propulsion.k
  Multiply : Product
  Power : Math  Operator=pow  SaturateOnIntegerOverflow=on
  cStar : Outport
  wires:
  Divide/1 -> cStar/1
  Gain/1 -> Divide/2
  Multiply/1 -> Divide/1
  speedOfSound/1 -> Multiply/2
  Combustion Efficiency/1 -> Multiply/1
  Power/1 -> Gain/1
  Divide1/1 -> Power/1
  Divide2/1 -> Power/2
  Combustion Efficiency1/1 -> Divide2/1, Divide1/2
  Combustion Efficiency2/1 -> Divide2/2
  Constant/1 -> Divide1/1

== system elementsLibrary/HREV1/Nozzle/calc_speedOfSound ==
  Tc : Inport
  Constant : Constant  Value=propulsion.gasConst
  Constant1 : Constant  Value=propulsion.k
  Multiply : Product  Inputs=3
  Sqrt : Sqrt  SaturateOnIntegerOverflow=on
  "speedOfSound " : Outport
  wires:
  Sqrt/1 -> "speedOfSound "/1
  Multiply/1 -> Sqrt/1
  Tc/1 -> Multiply/1
  Constant/1 -> Multiply/2
  Constant1/1 -> Multiply/3

== system elementsLibrary/HREV1/Nozzle/calc_thrust ==
  mdot_prop : Inport
  Ve_gas : Inport  Port=2
  Pe : Inport  Port=3
  Patm : Inport  Port=4
  Add : Sum
  Gain : Gain  Gain=propulsion.Ae
  Multiply : Product
  Subtract : Sum  Inputs=+-
  axialThrust : Outport
  wires:
  Add/1 -> axialThrust/1
  mdot_prop/1 -> Multiply/1
  Ve_gas/1 -> Multiply/2
  Multiply/1 -> Add/1
  Pe/1 -> Subtract/1
  Patm/1 -> Subtract/2
  Subtract/1 -> Gain/1
  Gain/1 -> Add/2

== system elementsLibrary/SingleChute/Rotational Motion/Subsystem ==
  ddtRiserLength : Inport
  RiserLength : Inport  Port=2
  Add : Sum
  Constant : Constant  Value=recovery.k_lines
  Constant1 : Constant  Value=recovery.c_lines
  Divide : Product  Inputs=/*
  Gain : Gain  Gain=-1
  Multiply : Product
  Multiply1 : Product
  Multiply2 : Product
  magnitude_1 : snippetLibrary/mathSnippets/magnitude_3
  magnitude_3 : snippetLibrary/mathSnippets/magnitude_3
  tensionP_E : Outport
  tensionR_E : Outport  Port=2
  wires:
  Constant/1 -> [K]
  [C] -> Multiply/1
  Constant1/1 -> [C]
  ddtRiserLength/1 -> magnitude_3/1
  RiserLength/1 -> magnitude_1/1, Divide/2
  [K] -> Multiply1/2
  magnitude_3/1 -> Multiply/2
  magnitude_1/1 -> Divide/1, Multiply1/1
  Multiply1/1 -> Add/2
  Multiply/1 -> Add/1
  Add/1 -> Multiply2/1
  Gain/1 -> tensionP_E/1
  Multiply2/1 -> tensionR_E/1, Gain/1
  Divide/1 -> Multiply2/2

== system elementsLibrary/SingleChute/Rotational Motion/calculate d//dt riser length ==
  ddtREP : Inport
  ddtRER : Inport  Port=2
  velocityP_E : Inport  Port=3
  velocityR_E : Inport  Port=4
  xBrid_P : Inport  Port=5
  xRoff_R : Inport  Port=6
  Add : Sum
  Add2 : Sum
  Matrix Multiply : Product  Multiplication=Matrix(*)
  Matrix Multiply1 : Product  Multiplication=Matrix(*)
  Subtract : Sum  Inputs=+-
  ddtRiserLength : Outport
  wires:
  Add/1 -> Subtract/1
  Matrix Multiply1/1 -> Add2/1
  Matrix Multiply/1 -> Add/2
  xRoff_R/1 -> Matrix Multiply1/2
  Subtract/1 -> ddtRiserLength/1  "ddtRiserLength"
  Add2/1 -> Subtract/2
  ddtREP/1 -> Matrix Multiply/1
  ddtRER/1 -> Matrix Multiply1/1
  velocityP_E/1 -> Add/1
  velocityR_E/1 -> Add2/2
  xBrid_P/1 -> Matrix Multiply/2

== system elementsLibrary/SingleChute/Rotational Motion/calculate rise length ==
  posP_E : Inport
  posR_E : Inport  Port=2
  REP : Inport  Port=3
  RER : Inport  Port=4
  XbridVector_B : Inport  Port=5
  XroffVector_B : Inport  Port=6
  Add : Sum
  Add2 : Sum
  Add3 : Sum  Inputs=+-
  Multiply : Product  Multiplication=Matrix(*)
  Multiply1 : Product  Multiplication=Matrix(*)
  riserLength_E : Outport
  wires:
  posR_E/1 -> Add2/2
  Add/1 -> Add3/1
  Add2/1 -> Add3/2
  Multiply1/1 -> Add2/1
  Multiply/1 -> Add/1
  posP_E/1 -> Add/2
  Add3/1 -> riserLength_E/1  "riserLength_E"
  XbridVector_B/1 -> Multiply/2
  REP/1 -> Multiply/1
  RER/1 -> Multiply1/1
  XroffVector_B/1 -> Multiply1/2

== system elementsLibrary/SingleChute/Rotational Motion/equations of rotational motion ==
  invREP : Inport
  tensionP_E : Inport  Port=2
  xBrid_P : Inport  Port=3
  xRoff_R : Inport  Port=4
  tensionR_E : Inport  Port=5
  invRER : Inport  Port=6
  angVelP : Inport  Port=7
  angVelR : Inport  Port=8
  Add : Sum  Inputs=-+
  Add1 : Sum  Inputs=-+
  Matrix Multiply{,1..3} (4 alike) : Product  Multiplication=Matrix(*)
  Multiply : Product  Multiplication=Matrix(*)
  Multiply1 : Product  Multiplication=Matrix(*)
  crossProduct{,1..3} (4 alike) : snippetLibrary/mathSnippets/crossProduct
  invInertia_Matrix_P : Subsystem
  invInertia_Matrix_R : Subsystem
  angularAcceleration_P : Outport
  angularAcceleration_R : Outport  Port=2
  wires:
  invInertia_Matrix_R/1(invInerMat) -> Matrix Multiply1/1
  Matrix Multiply/1 -> angularAcceleration_P/1  "angularAcceleration_P"
  Multiply/1 -> crossProduct2/2
  Matrix Multiply1/1 -> angularAcceleration_R/1  "angularAcceleration_R"
  Multiply1/1 -> crossProduct3/2
  xRoff_R/1 -> crossProduct3/1
  invInertia_Matrix_P/1(invInerMat) -> Matrix Multiply/1
  tensionP_E/1 -> Multiply/2
  invREP/1 -> Multiply/1
  xBrid_P/1 -> crossProduct2/1
  tensionR_E/1 -> Multiply1/2
  invRER/1 -> Multiply1/1
  invInertia_Matrix_P/2(inerMat) -> Matrix Multiply2/1
  angVelP/1 -> Matrix Multiply2/2, crossProduct/1
  Matrix Multiply2/1 -> crossProduct/2
  Add/1 -> Matrix Multiply/2
  crossProduct/1 -> Add/1
  crossProduct2/1 -> Add/2
  invInertia_Matrix_R/2(inerMat) -> Matrix Multiply3/1
  Add1/1 -> Matrix Multiply1/2
  Matrix Multiply3/1 -> crossProduct1/2
  crossProduct1/1 -> Add1/1
  angVelR/1 -> Matrix Multiply3/2, crossProduct1/1
  crossProduct3/1 -> Add1/2

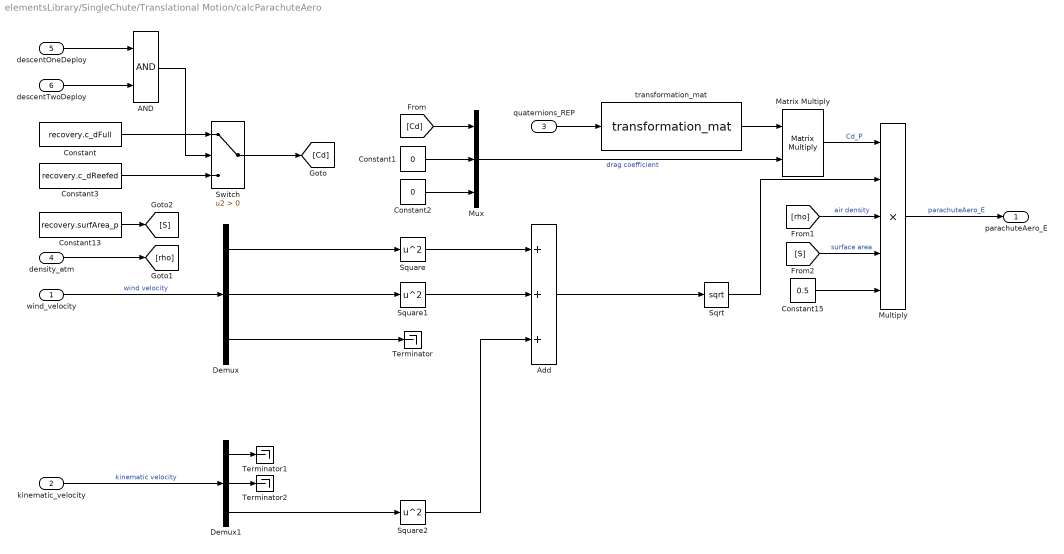
== system elementsLibrary/SingleChute/Translational Motion/calcParachuteAero  ==
  wind_velocity : Inport
  kinematic_velocity : Inport  Port=2
  quaternions_REP : Inport  Port=3
  density_atm : Inport  Port=4
  descentOneDeploy : Inport  Port=5
  descentTwoDeploy : Inport  Port=6
  AND : Logic  AllPortsSameDT=off  OutDataTypeStr=boolean
  Add : Sum  Inputs=+++
  Constant : Constant  Value=recovery.c_dFull
  Constant1 : Constant  Value=0
  Constant13 : Constant  Value=recovery.surfArea_p
  Constant15 : Constant  Value=0.5
  Constant2 : Constant  Value=0
  Constant3 : Constant  Value=recovery.c_dReefed
  Demux : Demux  Outputs=3
  Demux1 : Demux  Outputs=3
  Matrix Multiply : Product  Multiplication=Matrix(*)
  Multiply : Product  Inputs=5
  Mux : Mux  Inputs=3
  Sqrt : Sqrt  SaturateOnIntegerOverflow=on
  Square : Math  Operator=square  SaturateOnIntegerOverflow=on
  Square1 : Math  Operator=square  SaturateOnIntegerOverflow=on
  Square2 : Math  Operator=square  SaturateOnIntegerOverflow=on
  Switch : Switch  Criteria=u2 > Threshold
  Terminator : Terminator
  Terminator1 : Terminator
  Terminator2 : Terminator
  transformation_mat : snippetLibrary/mathSnippets/transformation_mat
  parachuteAero_E : Outport
  wires:
  Square2/1 -> Add/3
  Mux/1 -> Matrix Multiply/2  "drag coefficient"
  Square1/1 -> Add/2
  Constant1/1 -> Mux/2
  wind_velocity/1 -> Demux/1  "wind velocity"
  kinematic_velocity/1 -> Demux1/1  "kinematic velocity"
  [rho] -> Multiply/3  "air density"
  Square/1 -> Add/1
  Sqrt/1 -> Multiply/2
  Constant15/1 -> Multiply/5
  Demux/2 -> Square1/1
  [S] -> Multiply/4  "surface area"
  Demux/1 -> Square/1
  density_atm/1 -> [rho]
  [Cd] -> Mux/1
  Demux/3 -> Terminator/1
  Demux1/1 -> Terminator1/1
  Multiply/1 -> parachuteAero_E/1  "parachuteAero_E"
  Matrix Multiply/1 -> Multiply/1  "Cd_P"
  Demux1/3 -> Square2/1
  Add/1 -> Sqrt/1
  Constant13/1 -> [S]
  Demux1/2 -> Terminator2/1
  Constant2/1 -> Mux/3
  descentOneDeploy/1 -> AND/1
  descentTwoDeploy/1 -> AND/2
  Switch/1 -> [Cd]
  Constant/1 -> Switch/1
  Constant3/1 -> Switch/3
  AND/1 -> Switch/2
  transformation_mat/1 -> Matrix Multiply/1
  quaternions_REP/1 -> transformation_mat/1

== system elementsLibrary/barrowmanExt/Center of Pressure/Calc Xcp fins ==
  Mach : Inport
  Add : Sum
  Constant : Constant  Value=aerodynamics.Xf
  If : If  IfExpression=u1 < 0.5  ElseIfExpressions=u1>2
  If Action Subsystem : Subsystem  TreatAsAtomicUnit=on
  If Action Subsystem1 : Subsystem  TreatAsAtomicUnit=on
  If Action Subsystem2 : Subsystem  TreatAsAtomicUnit=on
  Merge : Merge  Inputs=3
  Xcp_fins : Outport
  wires:
  Mach/1 -> If Action Subsystem2/1(Mach), If Action Subsystem1/1(Mach), If/1
  If/1 -> If Action Subsystem/Action
  If Action Subsystem/1(Xcp_fins_subMach0.5) -> Merge/1
  Add/1 -> Xcp_fins/1
  Merge/1 -> Add/1
  Constant/1 -> Add/2
  If/2 -> If Action Subsystem1/Action
  If Action Subsystem1/1(Xcp_fins_above2) -> Merge/2
  If/3 -> If Action Subsystem2/Action
  If Action Subsystem2/1(Xcp_finsTrans) -> Merge/3

== system elementsLibrary/barrowmanExt/Coeff multiplier/magnitude_3 ==
  vector : Inport
  Add : Sum  Inputs=3
  Demux : Demux  Outputs=3
  Sqrt : Sqrt  SaturateOnIntegerOverflow=on
  Square : Math  Operator=square  SaturateOnIntegerOverflow=on
  magnitude : Outport
  wires:
  Sqrt/1 -> magnitude/1
  Add/1 -> Sqrt/1
  Demux/3 -> Add/3
  Demux/2 -> Add/2
  Demux/1 -> Add/1
  Square/1 -> Demux/1
  vector/1 -> Square/1

== system elementsLibrary/barrowmanExt/Coeff multiplier1/magnitude_3 ==
  vector : Inport
  Add : Sum  Inputs=3
  Demux : Demux  Outputs=3
  Sqrt : Sqrt  SaturateOnIntegerOverflow=on
  Square : Math  Operator=square  SaturateOnIntegerOverflow=on
  magnitude : Outport
  wires:
  Sqrt/1 -> magnitude/1
  Add/1 -> Sqrt/1
  Demux/3 -> Add/3
  Demux/2 -> Add/2
  Demux/1 -> Add/1
  Square/1 -> Demux/1
  vector/1 -> Square/1

== system elementsLibrary/barrowmanExt/Coefficent of drag 0 AOA/Base Drag Coefficient ==
  Mach : Inport
  MATLAB Function1 : MATLAB Function  TreatAsAtomicUnit=on
  Cd_Base : Outport
  wires:
  Mach/1 -> MATLAB Function1/1(mach)
  MATLAB Function1/1(baseD) -> Cd_Base/1

== system elementsLibrary/barrowmanExt/Coefficent of drag 0 AOA/Friction Drag Coefficient ==
  mach : Inport
  RE_Body : Inport  Port=2
  RE_Fins : Inport  Port=3
  ADD PARAMETER FOR NUM FINS : Constant  Value=aerodynamics.nf
  Add{,1..3} (4 alike) : Sum
  Constant : Constant  Value=aerodynamics.A_bwt
  Constant1 : Constant  Value=aerodynamics.l_TR  VectorParams1D=off  SampleTime=-1
  Constant10 : Constant  Value=2
  Constant11 : Constant  Value=aerodynamics.A_fp
  Constant12 : Constant  Value=aerodynamics.Ar
  Constant2 : Constant  Value=aerodynamics.dn
  Constant3 : Constant  Value=0.0001
  Constant4 : Constant  Value=4
  Constant5 : Constant
  Constant6 : Constant  Value=2
  Constant7 : Constant  Value=aerodynamics.tf
  Constant8 : Constant  Value=aerodynamics.lm
  Constant9 : Constant
  Divide : Product  Inputs=*//  SaturateOnIntegerOverflow=on  RndMeth=Zero
  Divide1 : Product  Inputs=**/
  Divide2 : Product  Inputs=*/
  MATLAB Function1 : MATLAB Function  TreatAsAtomicUnit=on
  MATLAB Function2 : MATLAB Function  TreatAsAtomicUnit=on
  Multiply : Product
  Multiply1 : Product
  Multiply2 : Product  Inputs=5
  CD_Friction : Outport
  wires:
  Divide2/1 -> CD_Friction/1
  Constant12/1 -> Divide2/2
  Add3/1 -> Divide2/1
  Multiply1/1 -> Add3/1
  Multiply2/1 -> Add3/2
  Constant11/1 -> Multiply2/5
  Add2/1 -> Multiply2/4
  Constant10/1 -> Multiply2/3
  ADD PARAMETER FOR NUM FINS/1 -> Multiply2/2
  MATLAB Function2/1(Cf) -> Multiply2/1
  Divide1/1 -> Add2/1
  Constant9/1 -> Add2/2
  Constant8/1 -> Divide1/3
  Constant6/1 -> Divide1/1
  Constant7/1 -> Divide1/2
  Add1/1 -> Multiply1/1
  Multiply/1 -> Multiply1/2
  Constant5/1 -> Add1/2
  Divide/1 -> Add1/1
  Add/1 -> Divide/3
  Constant2/1 -> Divide/1
  Constant4/1 -> Divide/2
  Constant3/1 -> Add/2
  Constant1/1 -> Add/1
  Constant/1 -> Multiply/1
  MATLAB Function1/1(Cf) -> Multiply/2
  mach/1 -> MATLAB Function1/1(mach), MATLAB Function2/1(mach)
  RE_Body/1 -> MATLAB Function1/2(RE)
  RE_Fins/1 -> MATLAB Function2/2(RE)

== system elementsLibrary/barrowmanExt/Coefficent of drag 0 AOA/Pressure Drag Coefficient ==
  Cd_Base : Inport
  mach : Inport  Port=2
  1-D Lookup Table : Lookup_n-D  NumberOfTableDimensions=1  BreakpointsForDimension1=aerodynamics.noseconePDBreakpoints  Table=aerodynamics.noseconePDTable  ExtrapMethod=Clip  UseLastTableValue=on  InternalRulePriority=Speed  RndMeth=Simplest  InputSameDT=on
  Add : Sum
  Fin Pressure Drag : Subsystem
  MATLAB Function : MATLAB Function  TreatAsAtomicUnit=on
  Cd_Pressure : Outport
  wires:
  Add/1 -> Cd_Pressure/1
  Fin Pressure Drag/1(finPD) -> Add/2
  1-D Lookup Table/1 -> Add/1
  Cd_Base/1 -> Fin Pressure Drag/2(baseD)
  MATLAB Function/1(stagD) -> Fin Pressure Drag/1(stagD)
  mach/1 -> 1-D Lookup Table/1, MATLAB Function/1(mach)

== system elementsLibrary/barrowmanExt/Coefficient of Axial Force/If Action Subsystem ==
  AOA : Inport
  Action Port : ActionPort
  Polynomial : Polyval  Coefs=aerodynamics.axialPolyLow
  Ax_multi : Outport
  wires:
  AOA/1 -> Polynomial/1
  Polynomial/1 -> Ax_multi/1

== system elementsLibrary/barrowmanExt/Coefficient of Axial Force/If Action Subsystem1 ==
  AOA_init : Inport
  Action Port : ActionPort
  Pi : Constant  Value=pi
  Subtract : Sum  Inputs=+-
  AOA : Outport
  wires:
  AOA_init/1 -> Subtract/2
  Pi/1 -> Subtract/1
  Subtract/1 -> AOA/1

== system elementsLibrary/barrowmanExt/Coefficient of Axial Force/If Action Subsystem2 ==
  AOA_init : Inport
  Action Port : ActionPort
  AOA : Outport
  wires:
  AOA_init/1 -> AOA/1

== system elementsLibrary/barrowmanExt/Coefficient of Axial Force/If Action Subsystem3 ==
  AOA : Inport
  Action Port : ActionPort
  Polynomial : Polyval  Coefs=aerodynamics.axialPolyHigh
  Ax_multi : Outport
  wires:
  AOA/1 -> Polynomial/1
  Polynomial/1 -> Ax_multi/1

== system elementsLibrary/barrowmanExt/Coefficient of Axial Force/If Action Subsystem4 ==
  Ax_multi_init : Inport
  Action Port : ActionPort
  Constant : Constant  Value=-1
  Multiply : Product
  Ax_multi : Outport
  wires:
  Ax_multi_init/1 -> Multiply/1
  Constant/1 -> Multiply/2
  Multiply/1 -> Ax_multi/1

== system elementsLibrary/barrowmanExt/Coefficient of Axial Force/If Action Subsystem5 ==
  Ax_multi_init : Inport
  Action Port : ActionPort
  Ax_multi : Outport
  wires:
  Ax_multi_init/1 -> Ax_multi/1
